simulink library "XXCopter"  (R2015a)
settings: Solver=ode45  StartTime=0.0  StopTime=10.0  RelTol=1e-3
undefined symbols (not defined in the file): a, C_d0, h, h_FA, h_M, I_prop, I_tube, inertia_switch, Initial_Omegas, Initial_Torques, J_FA, J_T, l, l_arm, m_FA, m_M, m_prop, Motor, Newton, Omega_TTO, Prop, R, Raphson, rho, Rotation_sign, sigma, tau, Tau_motors, theta_0, theta_1, Throtle_TTO, Torque_TTO, v_i0, v_i_adim, Vx_adim, Vz_adim
libraries: XXCopter x7, vrlib x5, XXCopter_C x3
settings Model: Creator=David  LastModifiedBy=David
settings OptimizationCC: ExpressionDepthLimit=2147483647
settings DebuggingCC: UnderspecifiedInitializationDetection=Classic  MergeDetectMultiDrivingBlocksExec=none  SolverPrmCheckMsg=warning  StateNameClashWarn=warning

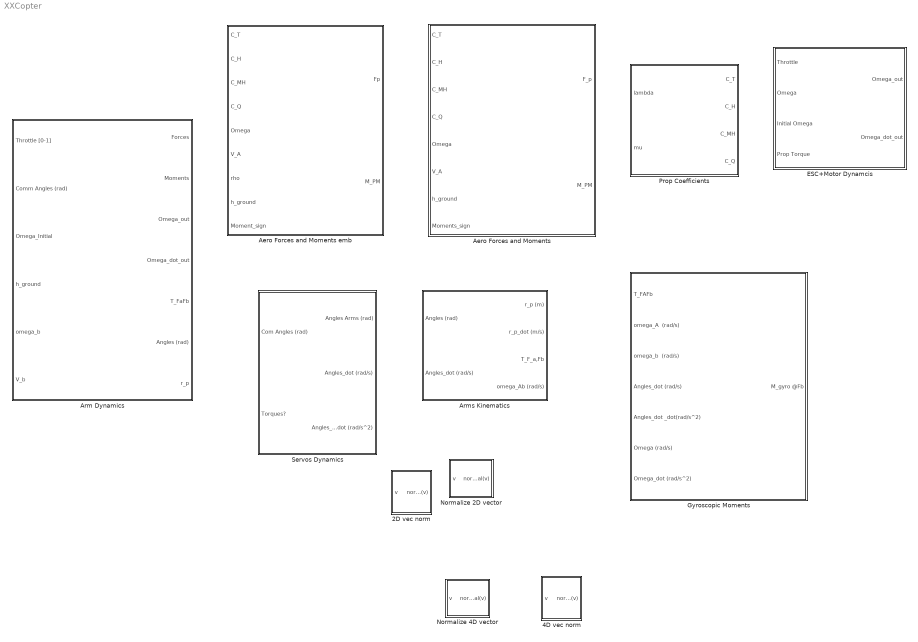
== system XXCopter ==
  2D vec norm : Subsystem  TreatAsAtomicUnit=on
  4D vec norm : Subsystem  TreatAsAtomicUnit=on
  Aero Forces and Moments : MATLAB Function  TreatAsAtomicUnit=on
  Aero Forces and Moments emb : Subsystem  TreatAsAtomicUnit=on
  Arm Dynamics : Subsystem  TreatAsAtomicUnit=on  mask(Arm dynamics, kinematics, forces and moments){Rot_sign=Rotation_sign(1), tau=Tau_motors, arm_hub_pos=l*[1;0;0], arm_axis=[l_arm;0;0], arm_num=1, eta_dir=[1;0;0], gamma_dir=[0;1;0], J_T=J_T, J_FA=J_FA, h=h, Torq_ini=Initial_Torques(1), Omega_ini=Initial_Omegas(1), init_eta=0, init_gamma=0, omega_n=35, xi=1.45, c=0}
      mask prompts: Rot_sign "Rotation sign"; tau "Tau motors"; arm_hub_pos "Arm Hub position"; arm_axis "Arm Hub from servo"; arm_num "Arm number"; eta_dir "eta direcction"; gamma_dir "gamma direction"; J_T "Inertia Motor+prop"; J_FA "Inertia Forearm"; h "h propeller hub"; Torq_ini "Torque Initial Condition"; Omega_ini "Omega Initial Condition"; init_eta "Initial eta  (rad)"; init_gamma "Initial gamma  (rad)"; omega_n "Servo natural frequency"; xi "Servo damping"; c "Derivative param"
      mask help:
      | This block only accepts arms oriented in x-axis or y-axis: eta and gamma directions can only be [1,0,0] or [0,1,0]
      | Note rotations order is [eta (pan) ,gamma (tilt),0]
      |
      | If Arm number 1 (Forward one)
      | eta_dir=[1,0,0]
      | gamma_dir=[0,1,0]
      |
      | If Arm number 2 or 3 (rear ones)
      | eta_dir=[0,1,0]
      | gamma_dir=[1,0,0]
      mask TypeOptions Rot_sign: Aerodynamics Propeller/Rot_sign | Gyroscopic Moments/Rot_sign
      mask TypeOptions tau: ESC+Motor Dynamcis/tau
      mask TypeOptions arm_hub_pos: Arms Kinematics/Arm_hub_position
      mask TypeOptions arm_axis: Gyroscopic Moments/Arm_axis
      mask TypeOptions arm_num: Arms Kinematics/Arm_number
      mask TypeOptions eta_dir: Arms Kinematics/eta_dir | Gyroscopic Moments/eta_dir
      mask TypeOptions gamma_dir: Arms Kinematics/gamma_dir | Gyroscopic Moments/gamma_dir
      mask TypeOptions J_T: ESC+Motor Dynamcis/J_T | Gyroscopic Moments/J_T
      mask TypeOptions J_FA: Gyroscopic Moments/J_FA
      mask TypeOptions h: Arms Kinematics/h_prop
      mask TypeOptions Torq_ini: Initial_torque/X0
      mask TypeOptions Omega_ini: initial_omega/X0
      mask TypeOptions init_eta: Servos Dynamics/init_eta
      mask TypeOptions omega_n: Servos Dynamics/omega_n
      mask TypeOptions xi: Servos Dynamics/xi
      mask TypeOptions c: Servos Dynamics/derv_param
      mask Display:
      | % fprintf(' Arm number %i \n dynamics',arm_num)
      | 
      | 
      | disp(['{\bf \fontsize{16}',sprintf('Arm number\n\n'),num2str(arm_num),sprintf('\n\n Dynamics '),'}'], 'texmode','on');
  Arms Kinematics : Subsystem  TreatAsAtomicUnit=on  mask{Arm_number=1, Arm_hub_position=l*[1;0;0], eta_dir=[1;0;0], gamma_dir=[0;1;0], h_prop=h}
      mask prompts: Arm_number "Arm number (1,2 or 3)"; Arm_hub_position "Arm Hub position"; eta_dir "eta direcction"; gamma_dir "gamma diretion"; h_prop "h of propeller hub"
      mask help:
      | If Arm number 1 (Forward one)
      | eta_dir=[1,0,0]
      | gamma_dir=[0,1,0]
      |
      | If Arm number 2 or 3 (rear ones)
      | eta_dir=[0,1,0]
      | gamma_dir=[1,0,0]
      mask TypeOptions Arm_number: Arm_no/Value
      mask TypeOptions Arm_hub_position: Hub_position/Value
      mask TypeOptions eta_dir: eta_dir/Gain
      mask TypeOptions gamma_dir: gamma_dir/Gain
      mask TypeOptions h_prop: h arm/Value
  ESC+Motor Dynamcis : Subsystem  TreatAsAtomicUnit=on  mask{Inertia_swithc_var=Motor+Prop, J_T=J_T, tau=tau}
      mask prompts: Inertia_swithc_var "Which inertia to use?"; J_T "Inertia Motor+Prop"; tau "Tau motors"
      mask TypeOptions Inertia_swithc_var: None | Motor+Prop
      mask Callback Inertia_swithc_var:
      | val = get_param(gcb,'MaskValues');
      | % lower(val{1})
      | switch lower(val{1})
      |  case {'none'}
      |   inertia_switch=1;
      |  case {'motor+prop'}
      |   inertia_switch=2;
      | end
      mask TypeOptions J_T: Inertia of prop+motor/Value
      mask TypeOptions tau: Time constant motors/Value
  Gyroscopic Moments : Subsystem  TreatAsAtomicUnit=on  mask{Arm_axis=[l_arm;0;0], Rot_sign=Rotation_sign(1), eta_dir=[1;0;0], gamma_dir=[0;1;0], J_T=J_T, J_FA=J_FA}
      mask prompts: Arm_axis "Arm axis from Servo origin"; Rot_sign "Rotation sign"; eta_dir "eta direction"; gamma_dir "gamma direction"; J_T "Inertia Motor+Prop"; J_FA "Inertia Foreamr"
      mask TypeOptions Arm_axis: Hub_position/Value
      mask TypeOptions Rot_sign: Rotation_sign/Value | Rotation_sign1/Value
      mask TypeOptions eta_dir: eta_dir/Gain | eta_dir1/Gain
      mask TypeOptions gamma_dir: gamma_dir/Gain | gamma_dir1/Gain
      mask TypeOptions J_T: Propeller and motor inertia/Value | Propeller and motor inertia1/Value
      mask TypeOptions J_FA: Forearm Inertia/Value | Forearm Inertia1/Value
  Normalize 2D vector : Subsystem  TreatAsAtomicUnit=on
  Normalize 4D vector : Subsystem  TreatAsAtomicUnit=on
  Prop Coefficients : MATLAB Function  TreatAsAtomicUnit=on
  Servos Dynamics : Subsystem  TreatAsAtomicUnit=on  mask{omega_n=35, xi=1.42, derv_param=0, init_eta=0, init_gamma=0}
      mask prompts: omega_n "Servo natural freq (rad/s) omega_n"; xi "Servo damping xi"; derv_param "Derivative parameter"; init_eta "Initial eta (rad)"; init_gamma "Initial gamma (rad)"
      mask TypeOptions init_eta: init_eta/Value | init_eta1/Value
      mask TypeOptions init_gamma: init_gamma/Value | init_gamma1/Value

== system XXCopter/2D vec norm ==
  v : Inport
  norm^2rm : Subsystem  TreatAsAtomicUnit=on
  sqrt : Sqrt  AlgorithmType=Newton-Raphson  SaturateOnIntegerOverflow=on
  norm(v) : Outport
  wires:
  sqrt/1 -> norm(v)/1
  norm^2rm/1(norm(v)) -> sqrt/1
  v/1 -> norm^2rm/1(v)

== system XXCopter/4D vec norm ==
  v : Inport
  norm^2rm : Subsystem  TreatAsAtomicUnit=on
  sqrt : Sqrt  AlgorithmType=Newton-Raphson  SaturateOnIntegerOverflow=on
  norm(v) : Outport
  wires:
  sqrt/1 -> norm(v)/1
  norm^2rm/1(norm(v)) -> sqrt/1
  v/1 -> norm^2rm/1(v)

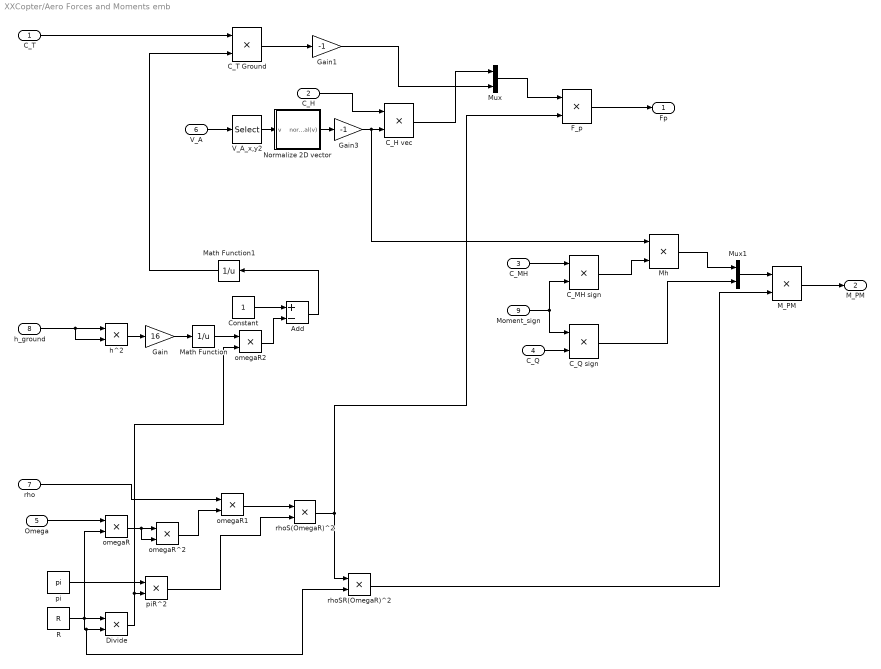
== system XXCopter/Aero Forces and Moments emb ==
  C_T : Inport
  C_H : Inport  Port=2
  C_MH : Inport  Port=3
  C_Q : Inport  Port=4
  Omega : Inport  Port=5
  V_A : Inport  Port=6
  rho : Inport  Port=7
  h_ground : Inport  Port=8
  Moment_sign : Inport  Port=9
  Add : Sum  Inputs=+-
  C_H vec : Product  Inputs=**
  C_MH sign : Product  Inputs=**
  C_Q sign : Product  Inputs=**
  C_T Ground : Product  Inputs=**
  Constant : Constant
  Divide : Product  Inputs=**
  F_p : Product  Inputs=**
  Gain : Gain  Gain=16
  Gain1 : Gain  Gain=-1
  Gain3 : Gain  Gain=-1
  M_PM : Product  Inputs=**
  Math Function : Math  Operator=reciprocal  SaturateOnIntegerOverflow=on
  Math Function1 : Math  Operator=reciprocal  SaturateOnIntegerOverflow=on
  Mh : Product  Inputs=**
  Mux : Mux  Inputs=[2,1]
  Mux1 : Mux  Inputs=[2,1]
  Normalize 2D vector : Subsystem  TreatAsAtomicUnit=on
  R : Constant  Value=R
  V_A_x,y2 : Selector  IndexMode=Zero-based  InputPortWidth=3  Indices=[0,1]
  h^2 : Product  Inputs=**
  omegaR : Product  Inputs=**
  omegaR1 : Product  Inputs=**
  omegaR2 : Product  Inputs=**
  omegaR^2 : Product  Inputs=**
  pi : Constant  Value=pi
  piR^2 : Product  Inputs=**
  rhoS(OmegaR)^2 : Product  Inputs=**
  rhoSR(OmegaR)^2 : Product  Inputs=**
  Fp : Outport
  "M_PM " : Outport  Port=2
  wires:
  M_PM/1 -> "M_PM "/1
  rhoSR(OmegaR)^2/1 -> M_PM/2
  C_Q sign/1 -> Mux1/2
  C_Q/1 -> C_Q sign/2
  Mux1/1 -> M_PM/1
  F_p/1 -> Fp/1
  Mh/1 -> Mux1/1
  C_MH sign/1 -> Mh/2
  Moment_sign/1 -> C_Q sign/1, C_MH sign/2
  C_MH/1 -> C_MH sign/1
  rhoS(OmegaR)^2/1 -> F_p/2, rhoSR(OmegaR)^2/1
  Mux/1 -> F_p/1
  Gain1/1 -> Mux/2
  C_H vec/1 -> Mux/1
  C_H/1 -> C_H vec/1
  Gain3/1 -> C_H vec/2, Mh/1
  Normalize 2D vector/1(normal(v)) -> Gain3/1
  V_A/1 -> V_A_x,y2/1
  V_A_x,y2/1 -> Normalize 2D vector/1(v)
  C_T Ground/1 -> Gain1/1
  Math Function1/1 -> C_T Ground/2
  Add/1 -> Math Function1/1
  omegaR2/1 -> Add/2
  Constant/1 -> Add/1
  Math Function/1 -> omegaR2/1
  Gain/1 -> Math Function/1
  h^2/1 -> Gain/1
  h_ground/1 -> h^2/1, h^2/2
  C_T/1 -> C_T Ground/1
  omegaR1/1 -> rhoS(OmegaR)^2/1
  piR^2/1 -> rhoS(OmegaR)^2/2
  omegaR^2/1 -> omegaR1/2
  omegaR/1 -> omegaR^2/1, omegaR^2/2
  rho/1 -> omegaR1/1
  Omega/1 -> omegaR/1
  Divide/1 -> piR^2/2, omegaR2/2
  pi/1 -> piR^2/1
  R/1 -> Divide/1, omegaR/2, Divide/2, rhoSR(OmegaR)^2/2

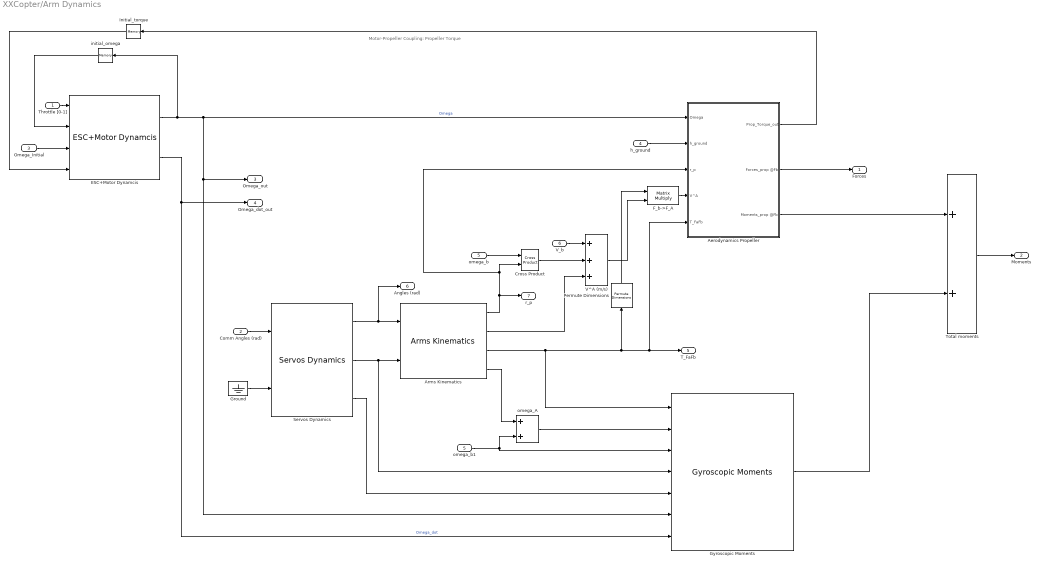
== system XXCopter/Arm Dynamics ==
  note: Motor-Propeller Coupling: Propeller Torque
  Throttle [0-1] : Inport
  Comm Angles (rad) : Inport  Port=2
  Omega_Initial : Inport  Port=3
  h_ground : Inport  Port=4
  omega_b : Inport  Port=5
  V_b : Inport  Port=6
  Aerodynamics Propeller : Subsystem  TreatAsAtomicUnit=on  mask{Rot_sign=Rot_sign}
      mask prompts: Rot_sign "Rotation Sign"
      settings: MinAlgLoopOccurrences=on
      mask TypeOptions Rot_sign: Rotation_sign/Value
  Arms Kinematics : XXCopter/Arms Kinematics  Arm_number=arm_num  Arm_hub_position=arm_hub_pos  eta_dir=eta_dir  gamma_dir=gamma_dir  h_prop=h
  Cross Product : vrlib/Utilities/Cross Product
  ESC+Motor Dynamcis : XXCopter/ESC+Motor Dynamcis  Inertia_swithc_var=Motor+Prop  J_T=J_T  tau=tau
  F_b->F_A : Product  Multiplication=Matrix(*)
  Ground : Ground
  Gyroscopic Moments : XXCopter/Gyroscopic Moments  Arm_axis=[l_arm;0;0]  Rot_sign=Rot_sign  eta_dir=eta_dir  gamma_dir=gamma_dir  J_T=J_T  J_FA=J_FA
  Initial_torque : Memory  X0=Torq_ini
  Permute Dimensions : PermuteDimensions
  Servos Dynamics : XXCopter/Servos Dynamics  omega_n=omega_n  xi=xi  derv_param=c  init_eta=init_eta  init_gamma=0
  Total moments : Sum
  V^A (m/s) : Sum  Inputs=+++
  initial_omega : Memory  X0=Omega_ini
  omega_A : Sum
  omega_b1 : InportShadow  Port=5
  Forces : Outport
  Moments : Outport  Port=2
  Omega_out : Outport  Port=3
  Omega_dot_out : Outport  Port=4
  T_FaFb : Outport  Port=5
  Angles (rad) : Outport  Port=6
  r_p : Outport  Port=7
  wires:
  Throttle [0-1]/1 -> ESC+Motor Dynamcis/1
  Omega_Initial/1 -> ESC+Motor Dynamcis/3
  ESC+Motor Dynamcis/2 -> Gyroscopic Moments/7, Omega_dot_out/1  "Omega_dot"
  ESC+Motor Dynamcis/1 -> initial_omega/1, Gyroscopic Moments/6, Omega_out/1, Aerodynamics Propeller/1(Omega)  "Omega"
  h_ground/1 -> Aerodynamics Propeller/2(h_ground)
  Comm Angles (rad)/1 -> Servos Dynamics/1
  Servos Dynamics/1 -> Arms Kinematics/1, Angles (rad)/1
  omega_b/1 -> Cross Product/1
  Cross Product/1 -> V^A (m/s)/2
  V_b/1 -> V^A (m/s)/1
  Arms Kinematics/2 -> V^A (m/s)/3
  Arms Kinematics/3 -> Gyroscopic Moments/1, Aerodynamics Propeller/5(T_FaFb), T_FaFb/1, Permute Dimensions/1
  Arms Kinematics/1 -> Aerodynamics Propeller/3(r_p), Cross Product/2, r_p/1
  Aerodynamics Propeller/2(Forces_prop @Fb) -> Forces/1
  Servos Dynamics/2 -> Gyroscopic Moments/4, Arms Kinematics/2
  Arms Kinematics/4 -> omega_A/1
  omega_b1/1 -> Gyroscopic Moments/3, omega_A/2
  omega_A/1 -> Gyroscopic Moments/2
  Servos Dynamics/3 -> Gyroscopic Moments/5
  Ground/1 -> Servos Dynamics/2
  Aerodynamics Propeller/3(Moments_prop @Fb) -> Total moments/1
  Gyroscopic Moments/1 -> Total moments/2
  Total moments/1 -> Moments/1
  Aerodynamics Propeller/1(Prop_Torque_out) -> Initial_torque/1
  Initial_torque/1 -> ESC+Motor Dynamcis/4
  initial_omega/1 -> ESC+Motor Dynamcis/2
  V^A (m/s)/1 -> F_b->F_A/2
  Permute Dimensions/1 -> F_b->F_A/1
  F_b->F_A/1 -> Aerodynamics Propeller/4(V^A)

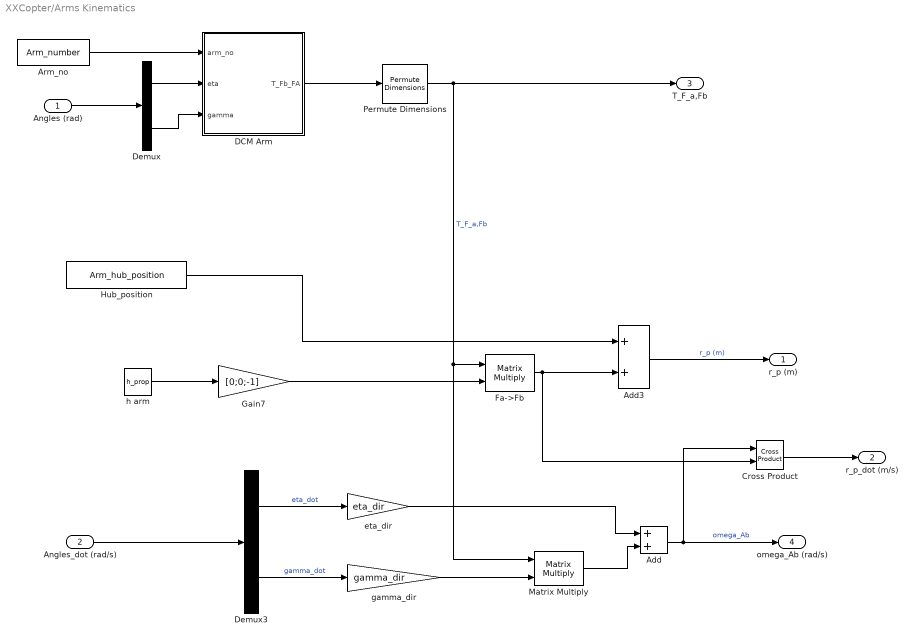
== system XXCopter/Arms Kinematics ==
  Angles (rad) : Inport
  Angles_dot (rad/s) : Inport  Port=2
  Add : Sum
  Add3 : Sum
  Arm_no : Constant  Value=Arm_number
  Cross Product : vrlib/Utilities/Cross Product
  DCM Arm : MATLAB Function  TreatAsAtomicUnit=on
  Demux : Demux  Outputs=2
  Demux3 : Demux  Outputs=2
  Fa->Fb : Product  Multiplication=Matrix(*)
  Gain7 : Gain  Gain=[0;0;-1]
  Hub_position : Constant  Value=Arm_hub_position
  Matrix Multiply : Product  Multiplication=Matrix(*)
  Permute Dimensions : PermuteDimensions
  eta_dir : Gain  Gain=eta_dir
  gamma_dir : Gain  Gain=gamma_dir
  h arm : Constant  Value=h_prop
  r_p (m) : Outport
  r_p_dot (m/s) : Outport  Port=2
  T_F_a,Fb : Outport  Port=3
  omega_Ab (rad/s) : Outport  Port=4
  wires:
  DCM Arm/1(T_Fb_FA) -> Permute Dimensions/1
  Permute Dimensions/1 -> T_F_a,Fb/1, Matrix Multiply/1, Fa->Fb/1  "T_F_a,Fb"
  Angles (rad)/1 -> Demux/1
  Demux/1 -> DCM Arm/2(eta)
  Demux/2 -> DCM Arm/3(gamma)
  Angles_dot (rad/s)/1 -> Demux3/1
  Demux3/2 -> gamma_dir/1  "gamma_dot"
  Demux3/1 -> eta_dir/1  "eta_dot"
  gamma_dir/1 -> Matrix Multiply/2
  Matrix Multiply/1 -> Add/2
  eta_dir/1 -> Add/1
  Add/1 -> Cross Product/1, omega_Ab (rad/s)/1  "omega_Ab"
  Add3/1 -> r_p (m)/1  "r_p (m)"
  h arm/1 -> Gain7/1
  Gain7/1 -> Fa->Fb/2
  Hub_position/1 -> Add3/1
  Fa->Fb/1 -> Cross Product/2, Add3/2
  Cross Product/1 -> r_p_dot (m/s)/1
  Arm_no/1 -> DCM Arm/1(arm_no)

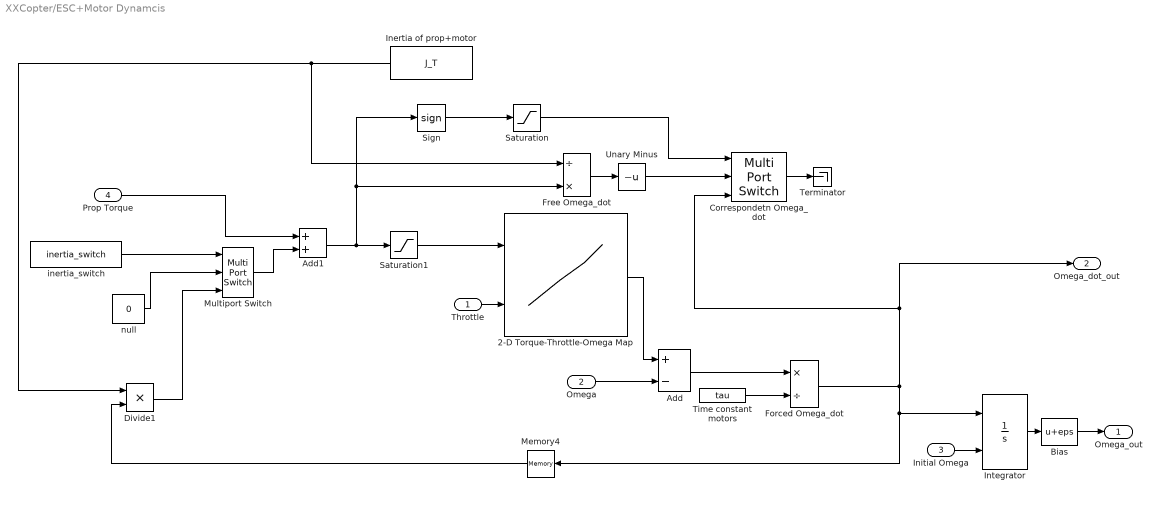
== system XXCopter/ESC+Motor Dynamcis ==
  Throttle : Inport
  Omega : Inport  Port=2
  Initial Omega : Inport  Port=3
  Prop Torque : Inport  Port=4
  2-D Torque-Throttle-Omega Map : Lookup_n-D  BreakpointsForDimension1=Torque_TTO(:,1)  BreakpointsForDimension2=Throtle_TTO(1,:)  Table=Omega_TTO  ExtrapMethod=Clip  DiagnosticForOutOfRangeInput=Warning  RemoveProtectionInput=on  RndMeth=Simplest  InputSameDT=on
  Add : Sum  Inputs=+-
  Add1 : Sum
  Bias : Bias  Bias=eps
  Correspondetn Omega_dot : MultiPortSwitch  DataPortOrder=Zero-based contiguous  Inputs=2
  Divide1 : Product  Inputs=**
  Forced Omega_dot : Product  Inputs=*/
  Free Omega_dot : Product  Inputs=/*
  Inertia of prop+motor : Constant  Value=J_T
  Integrator : Integrator  InitialConditionSource=external
  Memory4 : Memory
  Multiport Switch : MultiPortSwitch  Inputs=2
  Saturation : Saturate  UpperLimit=1  LowerLimit=0
  Saturation1 : Saturate  UpperLimit=inf  LowerLimit=0
  Sign : Signum
  Terminator : Terminator
  Time constant motors : Constant  Value=tau
  Unary Minus : UnaryMinus
  inertia_switch : Constant  Value=inertia_switch
  null : Constant  Value=0
  Omega_out : Outport
  Omega_dot_out : Outport  Port=2
  wires:
  Bias/1 -> Omega_out/1
  Divide1/1 -> Multiport Switch/3
  inertia_switch/1 -> Multiport Switch/1
  Memory4/1 -> Divide1/2
  Integrator/1 -> Bias/1
  Forced Omega_dot/1 -> Correspondetn Omega_dot/3, Omega_dot_out/1, Integrator/1, Memory4/1
  Add1/1 -> Sign/1, Free Omega_dot/2, Saturation1/1
  Throttle/1 -> 2-D Torque-Throttle-Omega Map/2
  null/1 -> Multiport Switch/2
  Inertia of prop+motor/1 -> Free Omega_dot/1, Divide1/1
  Multiport Switch/1 -> Add1/2
  Initial Omega/1 -> Integrator/2
  Time constant motors/1 -> Forced Omega_dot/2
  Add/1 -> Forced Omega_dot/1
  Omega/1 -> Add/2
  2-D Torque-Throttle-Omega Map/1 -> Add/1
  Prop Torque/1 -> Add1/1
  Free Omega_dot/1 -> Unary Minus/1
  Saturation/1 -> Correspondetn Omega_dot/1
  Sign/1 -> Saturation/1
  Unary Minus/1 -> Correspondetn Omega_dot/2
  Saturation1/1 -> 2-D Torque-Throttle-Omega Map/1
  Correspondetn Omega_dot/1 -> Terminator/1

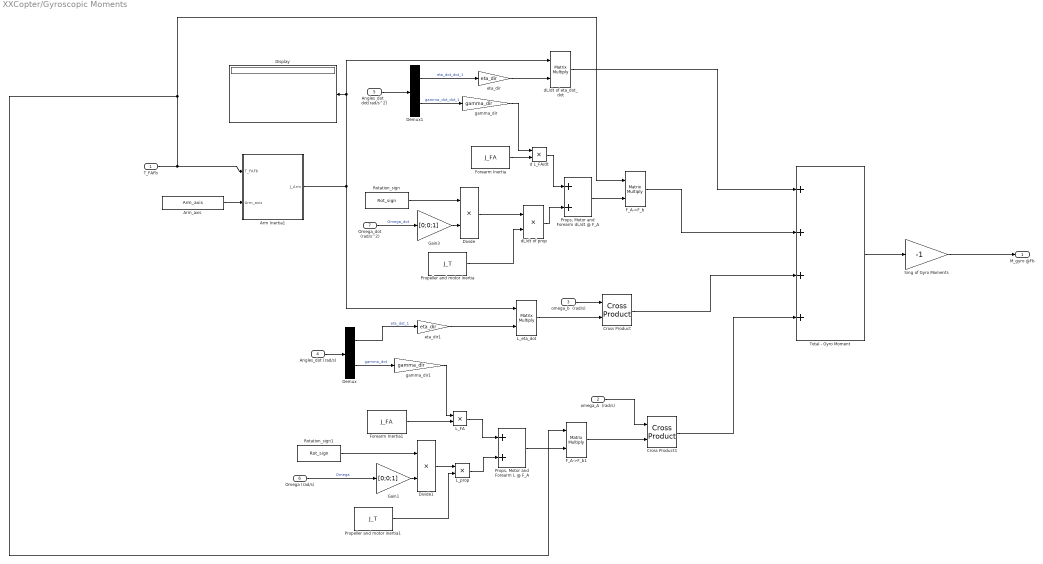
== system XXCopter/Gyroscopic Moments ==
  T_FAFb : Inport
  omega_A  (rad/s) : Inport  Port=2
  omega_b  (rad/s) : Inport  Port=3
  Angles_dot (rad/s) : Inport  Port=4
  Angles_dot _dot(rad/s^2) : Inport  Port=5
  Omega (rad/s) : Inport  Port=6
  Omega_dot (rad/s^2) : Inport  Port=7
  Arm Inertia1 : MATLAB Function  TreatAsAtomicUnit=on
  Arm_axis : Constant  Value=Arm_axis
  Cross Product : vrlib/Utilities/Cross Product
  Cross Product1 : vrlib/Utilities/Cross Product
  Demux : Demux  Outputs=2
  Demux1 : Demux  Outputs=2
  Display : Display
  Divide : Product  Inputs=**
  Divide1 : Product  Inputs=**
  F_A->F_b : Product  Multiplication=Matrix(*)
  F_A->F_b1 : Product  Multiplication=Matrix(*)
  Forearm Inertia : Constant  Value=J_FA
  Forearm Inertia1 : Constant  Value=J_FA
  Gain1 : Gain  Gain=[0;0;1]
  Gain3 : Gain  Gain=[0;0;1]
  L_FA : Product  Inputs=**
  L_eta_dot : Product  Multiplication=Matrix(*)
  L_prop : Product  Inputs=**
  Propeller and motor inertia : Constant  Value=J_T
  Propeller and motor inertia1 : Constant  Value=J_T
  "Props, Motor and Forearm L @ F_A" : Sum
  "Props, Motor and Forearm dL/dt @ F_A" : Sum
  Rotation_sign : Constant  Value=Rot_sign
  Rotation_sign1 : Constant  Value=Rot_sign
  Sing of Gyro Moments : Gain  Gain=-1
  Total - Gyro Moment : Sum  Inputs=++++
  d L_FA/dt : Product  Inputs=**
  dL/dt of eta_dot_dot : Product  Multiplication=Matrix(*)
  dL/dt of prop : Product  Inputs=**
  eta_dir : Gain  Gain=eta_dir
  eta_dir1 : Gain  Gain=eta_dir
  gamma_dir : Gain  Gain=gamma_dir
  gamma_dir1 : Gain  Gain=gamma_dir
  M_gyro @Fb : Outport
  wires:
  Gain1/1 -> Divide1/2
  Rotation_sign1/1 -> Divide1/1
  Gain3/1 -> Divide/2
  Rotation_sign/1 -> Divide/1
  Arm_axis/1 -> Arm Inertia1/2(Arm_axis)
  Sing of Gyro Moments/1 -> M_gyro @Fb/1
  Total - Gyro Moment/1 -> Sing of Gyro Moments/1
  Cross Product1/1 -> Total - Gyro Moment/4
  omega_A  (rad/s)/1 -> Cross Product1/1
  F_A->F_b1/1 -> Cross Product1/2
  T_FAFb/1 -> F_A->F_b1/1, F_A->F_b/1, Arm Inertia1/1(T_FAFb)
  "Props, Motor and Forearm L @ F_A"/1 -> F_A->F_b1/2
  Cross Product/1 -> Total - Gyro Moment/3
  dL/dt of eta_dot_dot/1 -> Total - Gyro Moment/1
  F_A->F_b/1 -> Total - Gyro Moment/2
  "Props, Motor and Forearm dL/dt @ F_A"/1 -> F_A->F_b/2
  Omega (rad/s)/1 -> Gain1/1  "Omega"
  L_prop/1 -> "Props, Motor and Forearm L @ F_A"/2
  L_FA/1 -> "Props, Motor and Forearm L @ F_A"/1
  Propeller and motor inertia1/1 -> L_prop/2
  Divide1/1 -> L_prop/1
  Forearm Inertia1/1 -> L_FA/2
  gamma_dir1/1 -> L_FA/1
  Demux/2 -> gamma_dir1/1  "gamma_dot"
  dL/dt of prop/1 -> "Props, Motor and Forearm dL/dt @ F_A"/2
  d L_FA/dt/1 -> "Props, Motor and Forearm dL/dt @ F_A"/1
  Propeller and motor inertia/1 -> dL/dt of prop/2
  Divide/1 -> dL/dt of prop/1
  Omega_dot (rad/s^2)/1 -> Gain3/1  "Omega_dot"
  Forearm Inertia/1 -> d L_FA/dt/2
  gamma_dir/1 -> d L_FA/dt/1
  Demux1/2 -> gamma_dir/1  "gamma_dot_dot_1"
  omega_b  (rad/s)/1 -> Cross Product/1
  L_eta_dot/1 -> Cross Product/2
  Demux/1 -> eta_dir1/1  "eta_dot_1"
  eta_dir1/1 -> L_eta_dot/2
  eta_dir/1 -> dL/dt of eta_dot_dot/2
  Arm Inertia1/1(J_Arm) -> L_eta_dot/1, dL/dt of eta_dot_dot/1, Display/1
  Demux1/1 -> eta_dir/1  "eta_dot_dot_1"
  Angles_dot _dot(rad/s^2)/1 -> Demux1/1
  Angles_dot (rad/s)/1 -> Demux/1

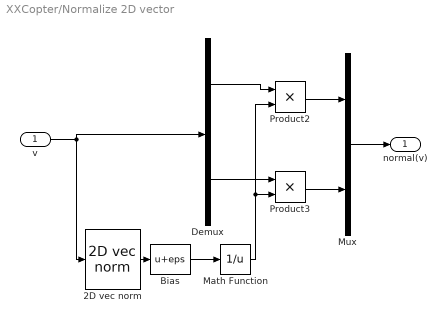
== system XXCopter/Normalize 2D vector ==
  v : Inport
  2D vec norm : XXCopter_C/2D vec norm
  Bias : Bias  Bias=eps
  Demux : Demux  Outputs=2
  Math Function : Math  Operator=reciprocal  SaturateOnIntegerOverflow=on
  Mux : Mux  Inputs=2
  Product2 : Product  Inputs=**
  Product3 : Product  Inputs=**
  normal(v) : Outport
  wires:
  Math Function/1 -> Product2/2, Product3/2
  Demux/2 -> Product3/1
  Demux/1 -> Product2/1
  Mux/1 -> normal(v)/1
  v/1 -> 2D vec norm/1, Demux/1
  Bias/1 -> Math Function/1
  Product2/1 -> Mux/1
  Product3/1 -> Mux/2
  2D vec norm/1 -> Bias/1

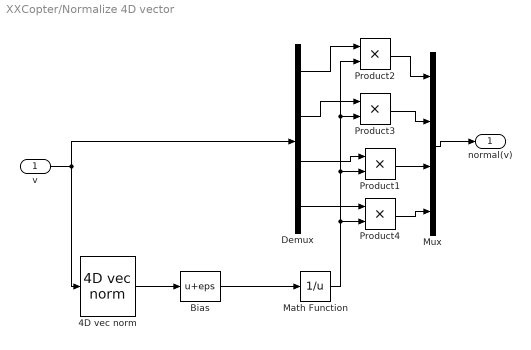
== system XXCopter/Normalize 4D vector ==
  v : Inport
  4D vec norm : XXCopter_C/4D vec norm
  Bias : Bias  Bias=eps
  Demux : Demux
  Math Function : Math  Operator=reciprocal  SaturateOnIntegerOverflow=on
  Mux : Mux
  Product{1..4} (4 alike) : Product  Inputs=**
  normal(v) : Outport
  wires:
  Product4/1 -> Mux/4
  Demux/4 -> Product4/1
  Demux/2 -> Product3/1
  Demux/1 -> Product2/1
  Mux/1 -> normal(v)/1
  v/1 -> Demux/1, 4D vec norm/1
  4D vec norm/1 -> Bias/1
  Product2/1 -> Mux/1
  Product3/1 -> Mux/2
  Demux/3 -> Product1/1
  Math Function/1 -> Product2/2, Product3/2, Product1/2, Product4/2
  Product1/1 -> Mux/3
  Bias/1 -> Math Function/1

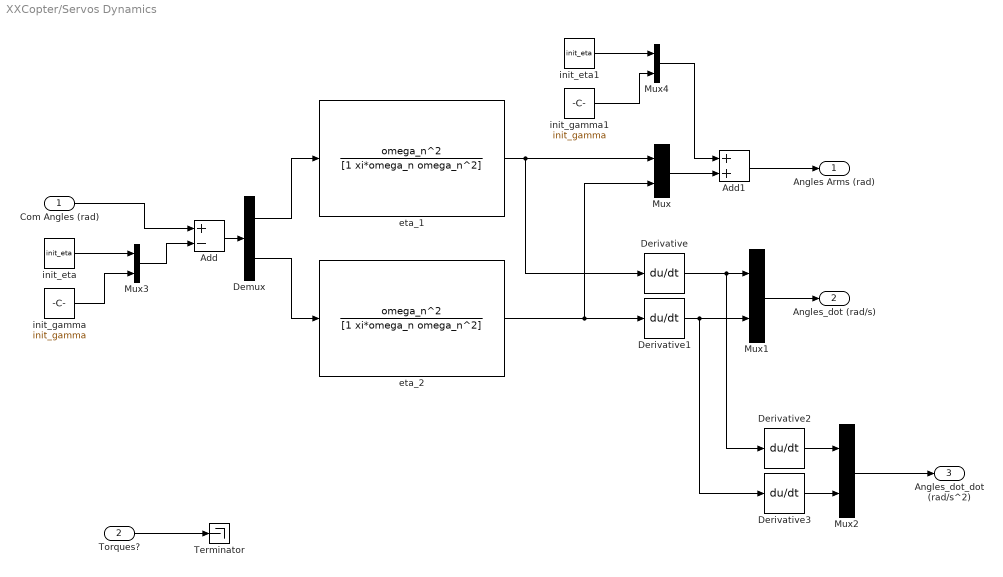
== system XXCopter/Servos Dynamics ==
  Com Angles (rad) : Inport
  Torques? : Inport  Port=2
  Add : Sum  Inputs=+-
  Add1 : Sum
  Demux : Demux  Outputs=2
  Derivative{,1..3} (4 alike) : Derivative  CoefficientInTFapproximation=derv_param
  Mux{,1..4} (5 alike) : Mux  Inputs=2
  Terminator : Terminator
  eta_1 : TransferFcn  Numerator=omega_n^2  Denominator=[1 xi*omega_n omega_n^2]
  eta_2 : TransferFcn  Numerator=omega_n^2  Denominator=[1 xi*omega_n omega_n^2]
  init_eta : Constant  Value=init_eta
  init_eta1 : Constant  Value=init_eta
  init_gamma : Constant  Value=init_gamma
  init_gamma1 : Constant  Value=init_gamma
  Angles Arms (rad) : Outport
  Angles_dot (rad/s) : Outport  Port=2
  Angles_dot_dot (rad/s^2) : Outport  Port=3
  wires:
  Com Angles (rad)/1 -> Add/1
  Demux/1 -> eta_1/1
  Demux/2 -> eta_2/1
  eta_1/1 -> Derivative/1, Mux/1
  eta_2/1 -> Mux/2, Derivative1/1
  Mux1/1 -> Angles_dot (rad/s)/1
  Mux2/1 -> Angles_dot_dot (rad/s^2)/1
  Derivative1/1 -> Derivative3/1, Mux1/2
  Derivative2/1 -> Mux2/1
  Derivative3/1 -> Mux2/2
  Derivative/1 -> Mux1/1, Derivative2/1
  Torques?/1 -> Terminator/1
  Add/1 -> Demux/1
  init_eta/1 -> Mux3/1
  Mux3/1 -> Add/2
  init_gamma/1 -> Mux3/2
  init_eta1/1 -> Mux4/1
  init_gamma1/1 -> Mux4/2
  Mux/1 -> Add1/2
  Mux4/1 -> Add1/1
  Add1/1 -> Angles Arms (rad)/1

== system XXCopter/2D vec norm/norm^2rm ==
  v : Inport
  Demux : Demux  Outputs=2
  Product : Product
  Product1 : Product
  Sum : Sum  Inputs=2
  norm(v) : Outport
  wires:
  v/1 -> Demux/1
  Sum/1 -> norm(v)/1
  Product/1 -> Sum/1
  Product1/1 -> Sum/2
  Demux/1 -> Product/1, Product/2
  Demux/2 -> Product1/2, Product1/1

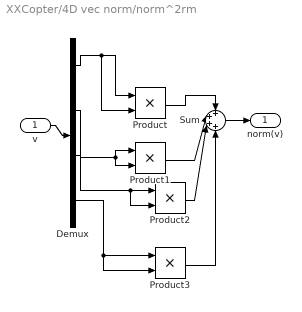
== system XXCopter/4D vec norm/norm^2rm ==
  v : Inport
  Demux : Demux
  Product{,1..3} (4 alike) : Product
  Sum : Sum  Inputs=4
  norm(v) : Outport
  wires:
  Product3/1 -> Sum/4
  Demux/4 -> Product3/1, Product3/2
  Product2/1 -> Sum/3
  Demux/3 -> Product2/1, Product2/2
  v/1 -> Demux/1
  Sum/1 -> norm(v)/1
  Product/1 -> Sum/1
  Product1/1 -> Sum/2
  Demux/1 -> Product/1, Product/2
  Demux/2 -> Product1/1, Product1/2

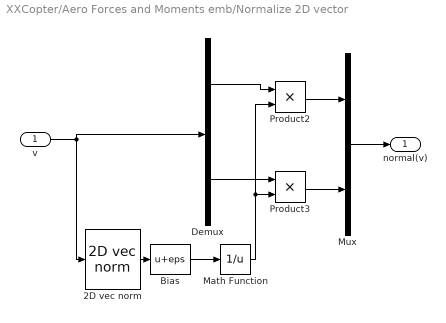
== system XXCopter/Aero Forces and Moments emb/Normalize 2D vector ==
  v : Inport
  2D vec norm : XXCopter_C/2D vec norm
  Bias : Bias  Bias=eps
  Demux : Demux  Outputs=2
  Math Function : Math  Operator=reciprocal  SaturateOnIntegerOverflow=on
  Mux : Mux  Inputs=2
  Product2 : Product  Inputs=**
  Product3 : Product  Inputs=**
  normal(v) : Outport
  wires:
  2D vec norm/1 -> Bias/1
  Product3/1 -> Mux/2
  Product2/1 -> Mux/1
  Bias/1 -> Math Function/1
  v/1 -> Demux/1, 2D vec norm/1
  Mux/1 -> normal(v)/1
  Demux/1 -> Product2/1
  Demux/2 -> Product3/1
  Math Function/1 -> Product3/2, Product2/2

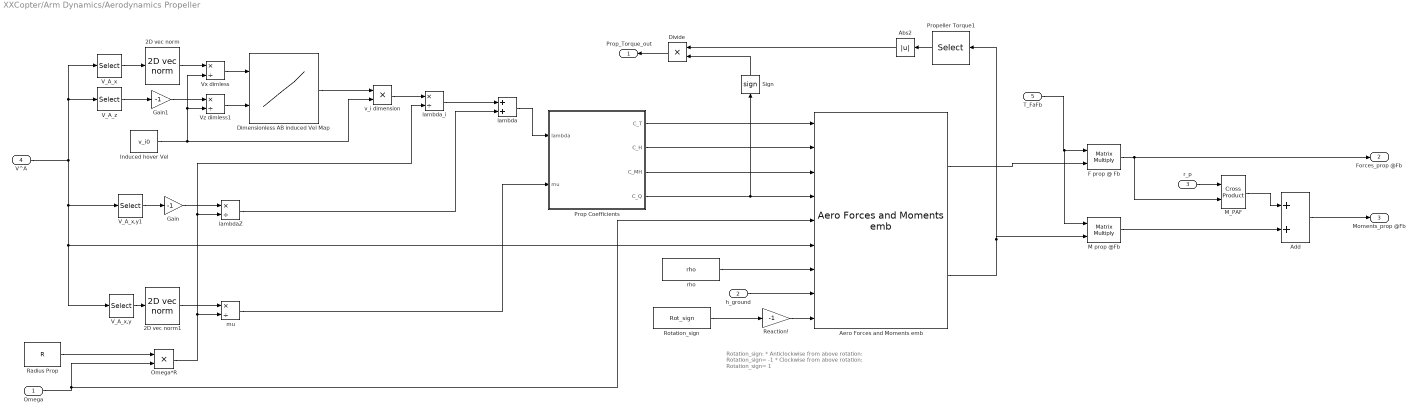
== system XXCopter/Arm Dynamics/Aerodynamics Propeller ==
  note: Rotation_sign:
      |
      | * Anticlockwise from above rotation: Rotation_sign= -1
      | * Clockwise from above rotation: Rotation_sign= 1
  Omega : Inport
  h_ground : Inport  Port=2
  r_p : Inport  Port=3
  V^A : Inport  Port=4
  T_FaFb : Inport  Port=5
  2D vec norm : XXCopter/2D vec norm
  2D vec norm1 : XXCopter/2D vec norm
  Abs2 : Abs
  Add : Sum
  Aero Forces and Moments emb : XXCopter/Aero Forces and Moments emb
  Dimensionless AB induced Vel Map : Lookup_n-D  BreakpointsForDimension1=Vx_adim  BreakpointsForDimension2=Vz_adim  BreakpointsForDimension3=[5, 7]  Table=v_i_adim  RndMeth=Simplest  InputSameDT=on
  Divide : Product  Inputs=**
  F prop @ Fb : Product  Multiplication=Matrix(*)
  Gain : Gain  Gain=-1
  Gain1 : Gain  Gain=-1
  Induced hover Vel : Constant  Value=v_i0
  M prop @Fb : Product  Multiplication=Matrix(*)
  M_PAF : vrlib/Utilities/Cross Product
  Omega*R : Product  Inputs=**
  Prop Coefficients : MATLAB Function  TreatAsAtomicUnit=on
  Propeller Torque1 : Selector  IndexMode=Zero-based  InputPortWidth=3  Indices=2
  Radius Prop : Constant  Value=R
  Reaction! : Gain  Gain=-1
  Rotation_sign : Constant  Value=Rot_sign
  Sign : Signum
  V_A_x : Selector  InputPortWidth=3  Indices=[1 2]
  V_A_x,y : Selector  InputPortWidth=3  Indices=[1 2]
  V_A_x,y1 : Selector  InputPortWidth=3  Indices=[3]
  V_A_z : Selector  InputPortWidth=3  Indices=3
  Vx dimless : Product  Inputs=*/
  Vz dimless1 : Product  Inputs=*/
  lambda : Sum
  lambdaZ : Product  Inputs=*/
  lambda_i : Product  Inputs=*/
  mu : Product  Inputs=*/
  rho : Constant  Value=rho
  v_i dimension : Product  Inputs=**
  Prop_Torque_out : Outport
  Forces_prop @Fb : Outport  Port=2
  Moments_prop @Fb : Outport  Port=3
  wires:
  Radius Prop/1 -> Omega*R/1
  V_A_x,y/1 -> 2D vec norm1/1
  2D vec norm1/1 -> mu/1
  Omega*R/1 -> mu/2, lambdaZ/2, lambda_i/2
  Vx dimless/1 -> Dimensionless AB induced Vel Map/1
  V_A_x/1 -> 2D vec norm/1
  Vz dimless1/1 -> Dimensionless AB induced Vel Map/2
  V_A_z/1 -> Gain1/1
  Induced hover Vel/1 -> v_i dimension/2, Vz dimless1/2, Vx dimless/2
  Dimensionless AB induced Vel Map/1 -> v_i dimension/1
  v_i dimension/1 -> lambda_i/1
  V_A_x,y1/1 -> Gain/1
  Gain/1 -> lambdaZ/1
  lambda_i/1 -> lambda/1
  lambdaZ/1 -> lambda/2
  Gain1/1 -> Vz dimless1/1
  lambda/1 -> Prop Coefficients/1(lambda)
  Prop Coefficients/1(C_T) -> Aero Forces and Moments emb/1
  Prop Coefficients/2(C_H) -> Aero Forces and Moments emb/2
  Prop Coefficients/3(C_MH) -> Aero Forces and Moments emb/3
  V^A/1 -> V_A_x,y/1, Aero Forces and Moments emb/6, V_A_x,y1/1, V_A_x/1, V_A_z/1
  Omega/1 -> Aero Forces and Moments emb/5, Omega*R/2
  Aero Forces and Moments emb/2 -> M prop @Fb/2, Propeller Torque1/1
  Add/1 -> Moments_prop @Fb/1
  h_ground/1 -> Aero Forces and Moments emb/8
  Rotation_sign/1 -> Reaction!/1
  T_FaFb/1 -> M prop @Fb/1, F prop @ Fb/1
  Aero Forces and Moments emb/1 -> F prop @ Fb/2
  F prop @ Fb/1 -> M_PAF/2, Forces_prop @Fb/1
  r_p/1 -> M_PAF/1
  M_PAF/1 -> Add/1
  M prop @Fb/1 -> Add/2
  2D vec norm/1 -> Vx dimless/1
  mu/1 -> Prop Coefficients/2(mu)
  Prop Coefficients/4(C_Q) -> Sign/1, Aero Forces and Moments emb/4
  Reaction!/1 -> Aero Forces and Moments emb/9
  rho/1 -> Aero Forces and Moments emb/7
  Divide/1 -> Prop_Torque_out/1
  Propeller Torque1/1 -> Abs2/1
  Sign/1 -> Divide/2
  Abs2/1 -> Divide/1

== matlab function XXCopter/Arm Dynamics/Aerodynamics Propeller/Prop Coefficients ==
  data: lambda input; C_T output; mu input; C_H output; C_MH output; C_Q output; sigma parameter; C_d0 parameter; a parameter; theta_0 parameter; theta_1 parameter
function [C_T,C_H,C_MH,C_Q] = Aero_coeff(lambda,mu, sigma, C_d0, a, theta_0, theta_1)

C_T = sigma*a/4*(theta_0*(2/3+mu^2) +theta_1/2*(1+mu^2) -  lambda );
C_Q =    +sigma*a/4*( 2/3*theta_0 - lambda + theta_1/2)*lambda + sigma*C_d0/8*(1+mu^2);   % Always positive!!!


C_H= sigma*a/4*mu*lambda*(theta_0+theta_1/2) + sigma*C_d0/4*mu; 
C_MH= sigma*a/4*( 2/3*theta_0*mu-1/2*lambda*mu+theta_1*mu/2  );

== matlab function XXCopter/Gyroscopic Moments/Arm Inertia1 ==
  data: T_FAFb input; Arm_axis input; J_Arm output; I_tube parameter; I_prop parameter; h_FA parameter; h_M parameter; m_FA parameter; m_M parameter; m_prop parameter; h parameter
function J_Arm  = Arm_inertia(T_FAFb,Arm_axis, I_tube, I_prop, h_FA, h_M, m_FA, m_M, m_prop, h)


r_FAO=Arm_axis+T_FAFb*[0;0;-h_FA];
r_MO=Arm_axis+T_FAFb*[0;0;-h_M];
r_po=Arm_axis+T_FAFb*[0;0;-h];

I_FA = m_FA*[ r_FAO(2)^2+r_FAO(3)^2,r_FAO(1)*r_FAO(2),r_FAO(1)*r_FAO(3);...
            r_FAO(1)*r_FAO(2), r_FAO(1)^2+r_FAO(3)^2, r_FAO(2)*r_FAO(3);...
            r_FAO(1)*r_FAO(3),r_FAO(2)*r_FAO(3), r_FAO(1)^2+r_FAO(2)^2];
I_M = m_M*[ r_MO(2)^2+r_MO(3)^2,r_MO(1)*r_MO(2),r_MO(1)*r_MO(3);...
            r_MO(1)*r_MO(2), r_MO(1)^2+r_MO(3)^2, r_MO(2)*r_MO(3);...
            r_MO(1)*r_MO(3),r_MO(2)*r_MO(3), r_MO(1)^2+r_MO(2)^2];
I_steiner = m_prop*[ r_po(2)^2+r_po(3)^2,r_po(1)*r_po(2),r_po(1)*r_po(3);...
            r_po(1)*r_po(2), r_po(1)^2+r_po(3)^2, r_po(2)*r_po(3);...
            r_po(1)*r_po(3),r_po(2)*r_po(3), r_po(1)^2+r_po(2)^2];


% J_Arm = T_FAFb*I_prop*T_FAFb'+ I_tube +I_FA+I_M+I_steiner;
J_Arm = T_FAFb*I_prop*T_FAFb' +I_FA+I_M+I_steiner; % Quitamos el tubo ya que es insignificante y hay que calcularlo para cada brazo

== matlab function XXCopter/Arms Kinematics/DCM Arm ==
  data: arm_no input; eta input; T_Fb_FA output; gamma input
function T_Fb_FA = DCM_Arm(arm_no,eta, gamma)
if arm_no==1
    T_Fb_FA = [ cos(gamma), sin(eta)*sin(gamma), -cos(eta)*sin(gamma);...
            0,cos(eta),sin(eta);...
            sin(gamma),-cos(gamma)*sin(eta),cos(gamma)*cos(eta) ];
elseif arm_no==2 || arm_no==3
    T_Fb_FA = [cos(eta),0,-sin(eta) ;...
            sin(eta)*sin(gamma),cos(gamma),cos(eta)*sin(gamma);...
            sin(eta)*cos(gamma),-sin(gamma),cos(eta)*cos(gamma)];
else
    error('That is not right: Chose a right arm'); 
end

== matlab function XXCopter/Aero Forces and Moments ==
  data: C_T input; C_H input; C_MH input; C_Q input; F_p output; M_PM output; Omega input; V_A input; h_ground input; Moments_sign input; R parameter; rho parameter
function [F_p,M_PM] = Aero_Forces_and_Moments(C_T,C_H,C_MH,C_Q,Omega,V_A,h_ground,Moments_sign, R, rho)



if V_A(1)==0 && V_A(2)==0
    H=[0;0];
else
    H=C_H*(-[V_A(1);V_A(2)])./norm([V_A(1);V_A(2)]);
end
%     C_T

T_temp=1/(1-R^2/(16*h_ground^2))*C_T;

F_p =   rho*pi*R^2*(Omega*R)^2*  [  H ; -T_temp ];
% pause

% Moments
% %     Moments_sign=1; % Anticlockwise from above
% %     Moments_sign=-1; % Clockwise from above 2y 4
if V_A(1)==0 && V_A(2)==0
    Mh=[0;0];
else
    Mh=Moments_sign*C_MH*(-[V_A(1);V_A(2)])./norm([V_A(1);V_A(2)]);% Note!!!! Signum of C_Mh depends on the spinning direction???
end

M_PM = rho*pi*R^3*(Omega*R)^2* [  Mh  ;  Moments_sign*C_Q ] ;

== matlab function XXCopter/Prop Coefficients ==
  data: lambda input; C_T output; mu input; C_H output; C_MH output; C_Q output; sigma parameter; C_d0 parameter; a parameter; theta_0 parameter; theta_1 parameter
function [C_T,C_H,C_MH,C_Q] = Aero_coeff(lambda,mu, sigma, C_d0, a, theta_0, theta_1)

C_T = sigma*a/4*(theta_0*(2/3+mu^2) +theta_1/2*(1+mu^2) -  lambda );
C_Q =    +sigma*a/4*( 2/3*theta_0 - lambda + theta_1/2)*lambda + sigma*C_d0/8*(1+mu^2);   % Always positive!!!


C_H= sigma*a/4*mu*lambda*(theta_0+theta_1/2) + sigma*C_d0/4*mu; 
C_MH= sigma*a/4*( 2/3*theta_0*mu-1/2*lambda*mu+theta_1*mu/2  );
